simulink model "error_space_model"  (R2024b)
settings: Solver=VariableStepAuto  StartTime=0.0  StopTime=10  RelTol=1e-3
values from neighbouring files (symbols this model uses):
  den_obs = [1, 2*wc_obs*delta_obs, wc_obs^2]    [error_space_script.m]
  K = Ke(2:end)    [conti_ss_script.m]    (also in discrete_script.m = Kdd; error_space_script.m = Kz(4:5); observer_script.m)
  Kz = place(Az, Bz, eigs)    [error_space_script.m]
  num_obs = [wc_obs^2, 0]    [error_space_script.m]
settings Model: Creator=pries  LastModifiedBy=pries

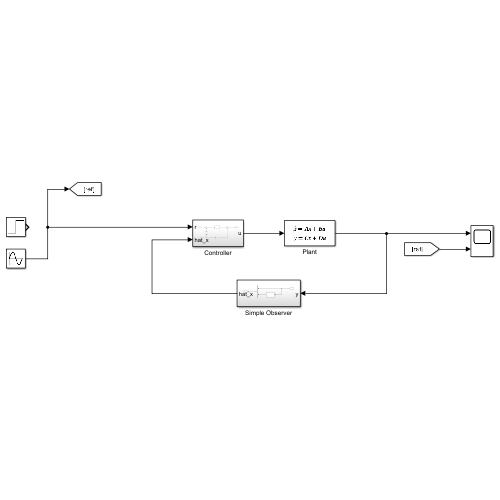
[thumbnail: Simulink's stored preview of the top-level diagram]
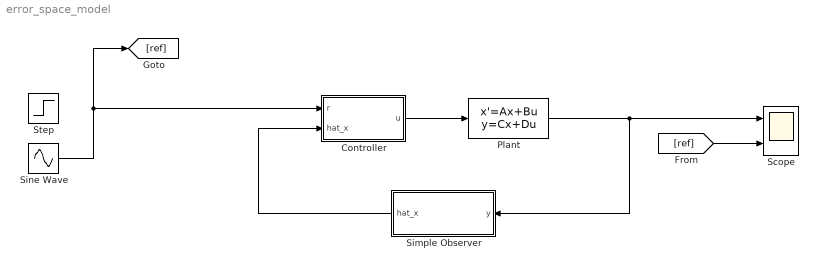
== system error_space_model ==
  Controller : Subsystem
  Plant : StateSpace  InitialCondition=0
  Scope : Scope  NumInputPorts=2
  Simple Observer : Subsystem
  Sine Wave : Sin  Frequency=6  SampleTime=0
  Step : Step  Time=0  SampleTime=0
  wires:
  Controller/1(u) -> Plant/1
  Simple Observer/1(hat_x) -> Controller/2(hat_x)
  Plant/1 -> Scope/1, Simple Observer/1(y)
  [ref] -> Scope/2
  Sine Wave/1 -> Controller/1(r), [ref]

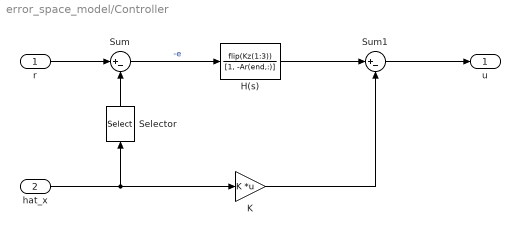
== system error_space_model/Controller ==
  r : Inport
  hat_x : Inport  Port=2
  H(s) : TransferFcn  Numerator=flip(Kz(1:3))  Denominator=[1, -Ar(end,:)]
  K : Gain  Gain=K  Multiplication=Matrix(K*u)
  Selector : Selector  InputPortWidth=2  IndexOptions=Index vector (dialog)  Indices=[1]  OutputSizes=1
  Sum : Sum  Inputs=|+-
  Sum1 : Sum  Inputs=|+-
  u : Outport
  wires:
  r/1 -> Sum/1
  Sum/1 -> H(s)/1  "-e"
  H(s)/1 -> Sum1/1
  Selector/1 -> Sum/2
  hat_x/1 -> K/1, Selector/1
  K/1 -> Sum1/2
  Sum1/1 -> u/1

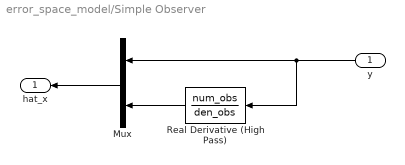
== system error_space_model/Simple Observer ==
  y : Inport
  Mux : Mux  Inputs=2
  Real Derivative (High Pass) : TransferFcn  Numerator=num_obs  Denominator=den_obs
  hat_x : Outport
  wires:
  Real Derivative (High Pass)/1 -> Mux/2
  y/1 -> Real Derivative (High Pass)/1, Mux/1
  Mux/1 -> hat_x/1
